simulink model "modelosimulinkparteB"  (R2018b)
settings: Solver=VariableStepAuto  StartTime=0.0  StopTime=400  RelTol=1e-3
settings Model: Creator=pedro  LastModifiedBy=XAVIER

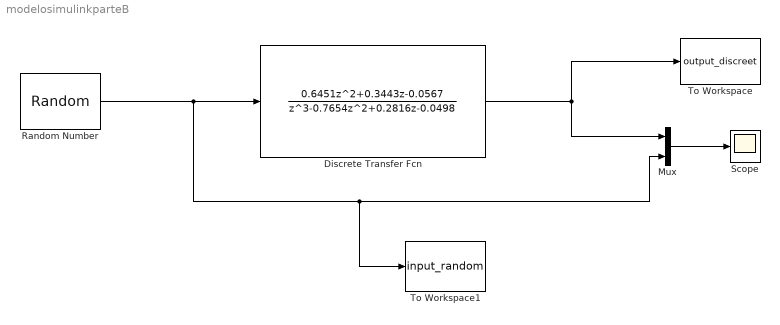
== system modelosimulinkparteB ==
  Discrete Transfer Fcn : DiscreteTransferFcn  Numerator=[0 0.6451 0.3443 -0.0567]  Denominator=[1.0000 -0.7654 0.2816 -0.0498]
  Mux : Mux  Inputs=2
  Random Number : RandomNumber  SampleTime=0.1
  Scope : Scope
  To Workspace : ToWorkspace  VariableName=output_discreet  SampleTime=-1
      settings: Save2DSignal=2-D array (concatenate along first dimension)
  To Workspace1 : ToWorkspace  VariableName=input_random  SampleTime=-1
      settings: Save2DSignal=2-D array (concatenate along first dimension)
  wires:
  Random Number/1 -> To Workspace1/1, Mux/2, Discrete Transfer Fcn/1
  Mux/1 -> Scope/1
  Discrete Transfer Fcn/1 -> Mux/1, To Workspace/1
